simulink library "EqM"  (R2024a)
settings: Solver=VariableStepAuto  StartTime=0.0  StopTime=10.0  RelTol=1e-3
values from neighbouring files (symbols this model uses):
  g = 9.80665    [Initialization.m]    (also in Initialization_alt2.m; Initialization_cg1.m; Initialization_loop.m; Initialization_v2.m)
libraries: $bdroot x1
settings Model: Creator=Caê  LastModifiedBy=Caê
settings RTWCC: GPUComputeCapability=3.5

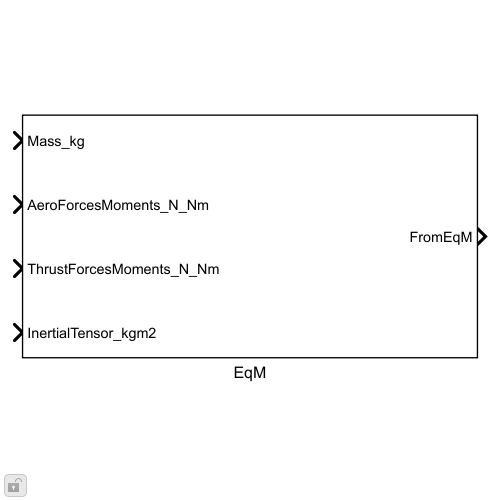
[thumbnail: Simulink's stored preview of the top-level diagram]
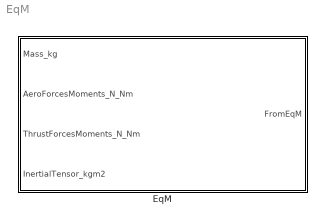
== system EqM ==
  EqM : Subsystem

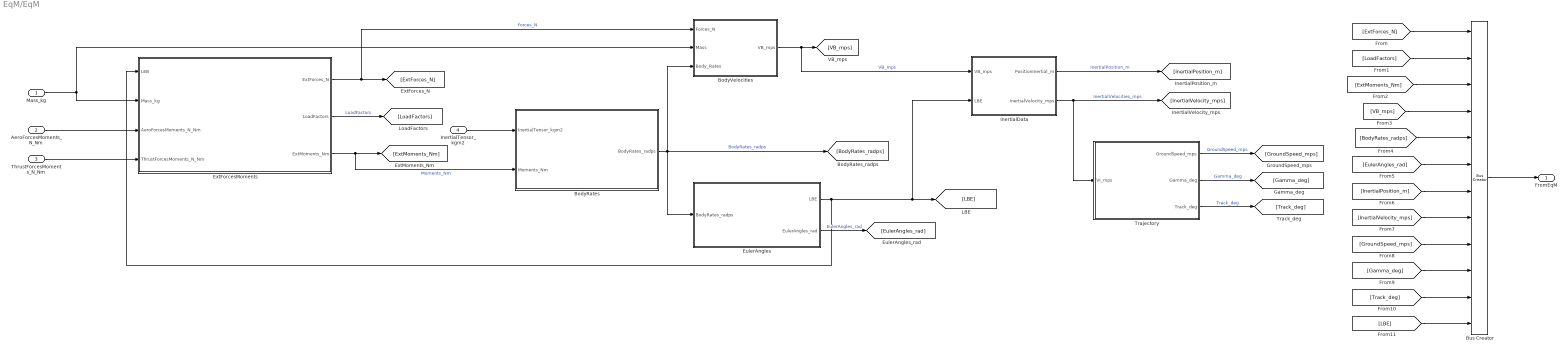
== system EqM/EqM ==
  Mass_kg : Inport
  AeroForcesMoments_N_Nm : Inport  Port=2
  ThrustForcesMoments_N_Nm : Inport  Port=3
  InertialTensor_kgm2 : Inport  Port=4
  BodyRates : Subsystem
  BodyVelocities : Subsystem
  Bus Creator : BusCreator  Inputs=12
  EulerAngles : Subsystem
  ExtForcesMoments : Subsystem
  InertialData : Subsystem
  Trajectory : Subsystem
  FromEqM : Outport
  wires:
  [LBE] -> Bus Creator/12
  [InertialPosition_m] -> Bus Creator/7
  ExtForcesMoments/3(ExtMoments_Nm) -> BodyRates/2(Moments_Nm), [ExtMoments_Nm]  "Moments_Nm"
  [EulerAngles_rad] -> Bus Creator/6
  [GroundSpeed_mps] -> Bus Creator/9
  Mass_kg/1 -> BodyVelocities/2(Mass), ExtForcesMoments/2(Mass_kg)
  ThrustForcesMoments_N_Nm/1 -> ExtForcesMoments/4(ThrustForcesMoments_N_Nm)
  InertialTensor_kgm2/1 -> BodyRates/1(InertialTensor_kgm2)
  [InertialVelocity_mps] -> Bus Creator/8
  [LoadFactors] -> Bus Creator/2
  InertialData/2(InertialVelocity_mps) -> [InertialVelocity_mps], Trajectory/1(VI_mps)  "InertialVelocities_mps"
  Bus Creator/1 -> FromEqM/1
  [BodyRates_radps] -> Bus Creator/5
  [Track_deg] -> Bus Creator/11
  EulerAngles/2(EulerAngles_rad) -> [EulerAngles_rad]  "EulerAngles_rad"
  [Gamma_deg] -> Bus Creator/10
  InertialData/1(PositionInertial_m) -> [InertialPosition_m]  "InertialPosition_m"
  ExtForcesMoments/2(LoadFactors) -> [LoadFactors]  "LoadFactors"
  BodyRates/1(BodyRates_radps) -> [BodyRates_radps], EulerAngles/1(BodyRates_radps), BodyVelocities/3(Body_Rates)  "BodyRates_radps"
  ExtForcesMoments/1(ExtForces_N) -> [ExtForces_N], BodyVelocities/1(Forces_N)  "Forces_N"
  BodyVelocities/1(VB_mps) -> [VB_mps], InertialData/1(VB_mps)  "VB_mps"
  [ExtMoments_Nm] -> Bus Creator/3
  AeroForcesMoments_N_Nm/1 -> ExtForcesMoments/3(AeroForcesMoments_N_Nm)
  Trajectory/1(GroundSpeed_mps) -> [GroundSpeed_mps]  "GroundSpeed_mps"
  [ExtForces_N] -> Bus Creator/1
  Trajectory/3(Track_deg) -> [Track_deg]  "Track_deg"
  EulerAngles/1(LBE) -> ExtForcesMoments/1(LEB), InertialData/2(LBE), [LBE]
  Trajectory/2(Gamma_deg) -> [Gamma_deg]  "Gamma_deg"
  [VB_mps] -> Bus Creator/4

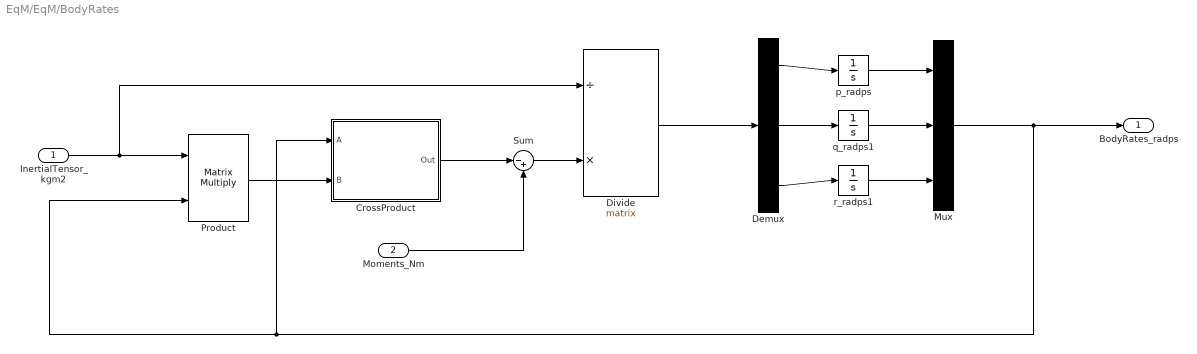
== system EqM/EqM/BodyRates ==
  InertialTensor_kgm2 : Inport
  Moments_Nm : Inport  Port=2
  CrossProduct : Subsystem
  Demux : Demux  Outputs=3
  Divide : Product  Inputs=/*  Multiplication=Matrix(*)
  Mux : Mux  Inputs=3
  Product : Product  Multiplication=Matrix(*)
  Sum : Sum  Inputs=|-+
  p_radps : Integrator  ContinuousStateAttributes='p_radps'
  q_radps1 : Integrator  ContinuousStateAttributes='q_radps'
  r_radps1 : Integrator  ContinuousStateAttributes='r_radps'
  BodyRates_radps : Outport
  wires:
  Demux/3 -> r_radps1/1
  InertialTensor_kgm2/1 -> Divide/1, Product/1
  Mux/1 -> BodyRates_radps/1, CrossProduct/1(A), Product/2
  q_radps1/1 -> Mux/2
  Sum/1 -> Divide/2
  Demux/1 -> p_radps/1
  Product/1 -> CrossProduct/2(B)
  p_radps/1 -> Mux/1
  CrossProduct/1(Out) -> Sum/1
  Moments_Nm/1 -> Sum/2
  r_radps1/1 -> Mux/3
  Demux/2 -> q_radps1/1
  Divide/1 -> Demux/1

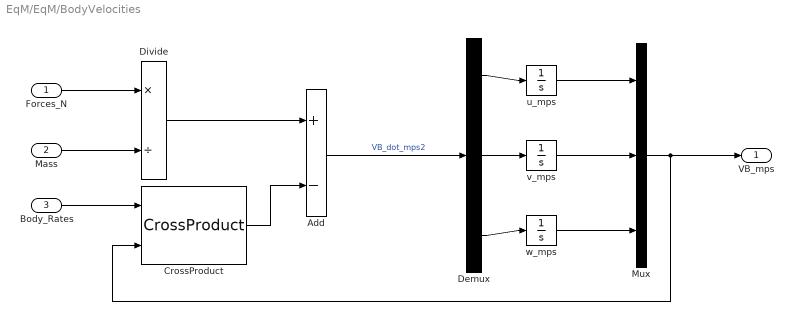
== system EqM/EqM/BodyVelocities ==
  Forces_N : Inport
  Mass : Inport  Port=2
  Body_Rates : Inport  Port=3
  Add : Sum  Inputs=+-
  CrossProduct : $bdroot/EqM/BodyRates/CrossProduct  SystemSampleTime=-1  VariantActivationTime=update diagram  AllowFlexibleInterface=on  Latency=0  AutoFrameSizeCalculation=off
  Demux : Demux  Outputs=3
  Divide : Product  Inputs=*/
  Mux : Mux  Inputs=3
  u_mps : Integrator  ContinuousStateAttributes='u_mps'
  v_mps : Integrator  ContinuousStateAttributes='v_mps'
  w_mps : Integrator  ContinuousStateAttributes='w_mps'
  VB_mps : Outport
  wires:
  CrossProduct/1 -> Add/2
  Demux/3 -> w_mps/1
  Mux/1 -> CrossProduct/2, VB_mps/1
  Forces_N/1 -> Divide/1
  Demux/2 -> v_mps/1
  u_mps/1 -> Mux/1
  Demux/1 -> u_mps/1
  Mass/1 -> Divide/2
  Body_Rates/1 -> CrossProduct/1
  Add/1 -> Demux/1  "VB_dot_mps2"
  w_mps/1 -> Mux/3
  v_mps/1 -> Mux/2
  Divide/1 -> Add/1

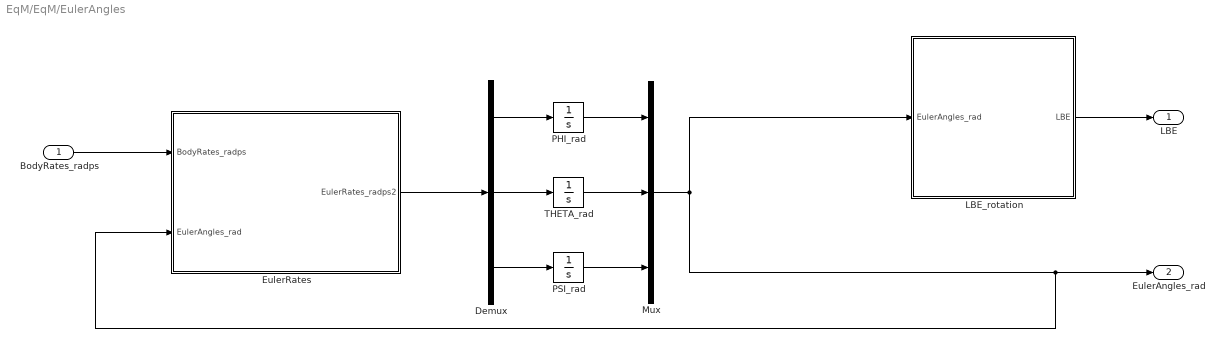
== system EqM/EqM/EulerAngles ==
  BodyRates_radps : Inport
  Demux : Demux  Outputs=3
  EulerRates : Subsystem
  LBE_rotation : Subsystem
  Mux : Mux  Inputs=3
  PHI_rad : Integrator  ContinuousStateAttributes='PHI_rad'
  PSI_rad : Integrator  ContinuousStateAttributes='PSI_rad'
  THETA_rad : Integrator  ContinuousStateAttributes='THETA_rad'
  LBE : Outport
  EulerAngles_rad : Outport  Port=2
  wires:
  Demux/3 -> PSI_rad/1
  Demux/2 -> THETA_rad/1
  Demux/1 -> PHI_rad/1
  PHI_rad/1 -> Mux/1
  Mux/1 -> EulerRates/2(EulerAngles_rad), EulerAngles_rad/1, LBE_rotation/1(EulerAngles_rad)
  PSI_rad/1 -> Mux/3
  EulerRates/1(EulerRates_radps2) -> Demux/1
  THETA_rad/1 -> Mux/2
  BodyRates_radps/1 -> EulerRates/1(BodyRates_radps)
  LBE_rotation/1(LBE) -> LBE/1

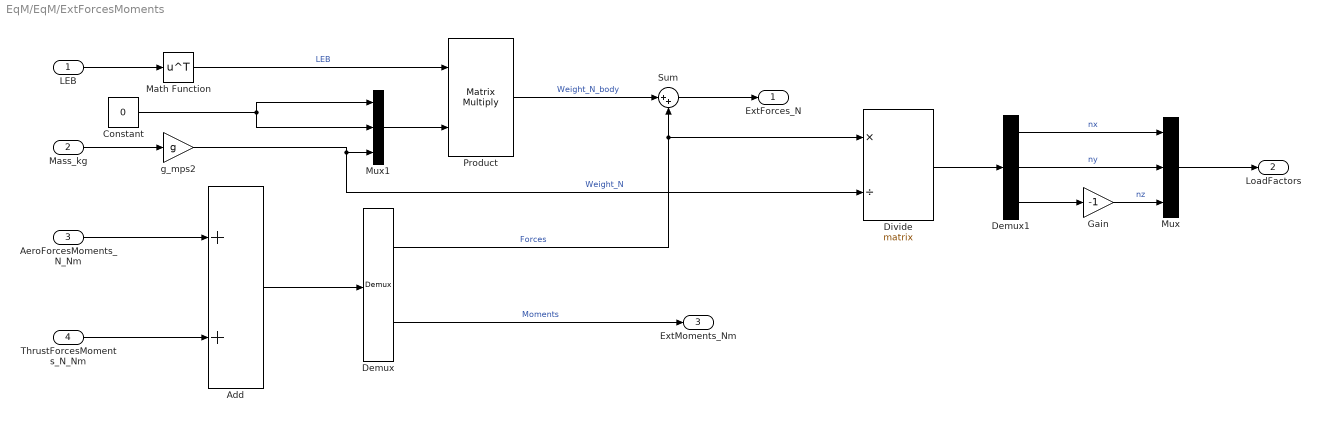
== system EqM/EqM/ExtForcesMoments ==
  LEB : Inport
  Mass_kg : Inport  Port=2
  AeroForcesMoments_N_Nm : Inport  Port=3
  ThrustForcesMoments_N_Nm : Inport  Port=4
  Add : Sum
  Constant : Constant  Value=0
  Demux : Demux  Outputs=2
  Demux1 : Demux  Outputs=3
  Divide : Product  Inputs=*/  Multiplication=Matrix(*)
  Gain : Gain  Gain=-1
  Math Function : Math  Operator=transpose
  Mux : Mux  Inputs=3
  Mux1 : Mux  Inputs=3
  Product : Product  Multiplication=Matrix(*)
  Sum : Sum  Inputs=|++
  g_mps2 : Gain  Gain=g
  ExtForces_N : Outport
  LoadFactors : Outport  Port=2
  ExtMoments_Nm : Outport  Port=3
  wires:
  Add/1 -> Demux/1
  Sum/1 -> ExtForces_N/1
  Mass_kg/1 -> g_mps2/1
  LEB/1 -> Math Function/1
  Demux/1 -> Divide/1, Sum/2  "Forces"
  Gain/1 -> Mux/3  "nz"
  Constant/1 -> Mux1/2, Mux1/1
  Math Function/1 -> Product/1  "LEB"
  g_mps2/1 -> Divide/2, Mux1/3  "Weight_N"
  Demux1/1 -> Mux/1  "nx"
  Product/1 -> Sum/1  "Weight_N_body"
  Demux1/2 -> Mux/2  "ny"
  Demux/2 -> ExtMoments_Nm/1  "Moments"
  Mux/1 -> LoadFactors/1
  AeroForcesMoments_N_Nm/1 -> Add/1
  Divide/1 -> Demux1/1
  ThrustForcesMoments_N_Nm/1 -> Add/2
  Demux1/3 -> Gain/1
  Mux1/1 -> Product/2

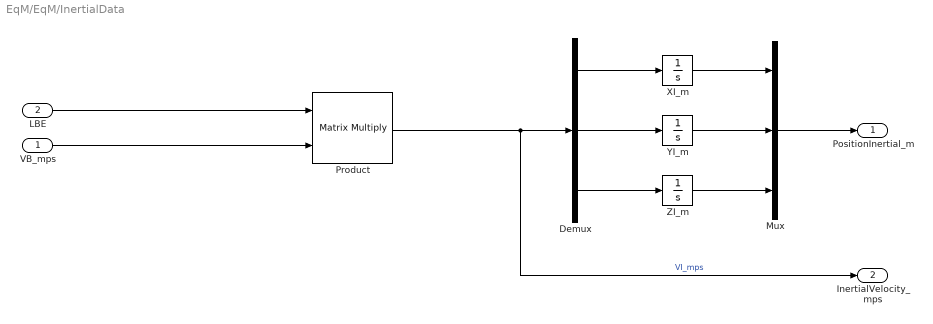
== system EqM/EqM/InertialData ==
  VB_mps : Inport
  LBE : Inport  Port=2
  Demux : Demux  Outputs=3
  Mux : Mux  Inputs=3
  Product : Product  Multiplication=Matrix(*)
  XI_m : Integrator  ContinuousStateAttributes='XI_m'
  YI_m : Integrator  ContinuousStateAttributes='YI_m'
  ZI_m : Integrator  ContinuousStateAttributes='ZI_m'
  PositionInertial_m : Outport
  InertialVelocity_mps : Outport  Port=2
  wires:
  Demux/1 -> XI_m/1
  ZI_m/1 -> Mux/3
  VB_mps/1 -> Product/2
  Product/1 -> InertialVelocity_mps/1, Demux/1  "VI_mps"
  XI_m/1 -> Mux/1
  Mux/1 -> PositionInertial_m/1
  YI_m/1 -> Mux/2
  Demux/3 -> ZI_m/1
  Demux/2 -> YI_m/1
  LBE/1 -> Product/1

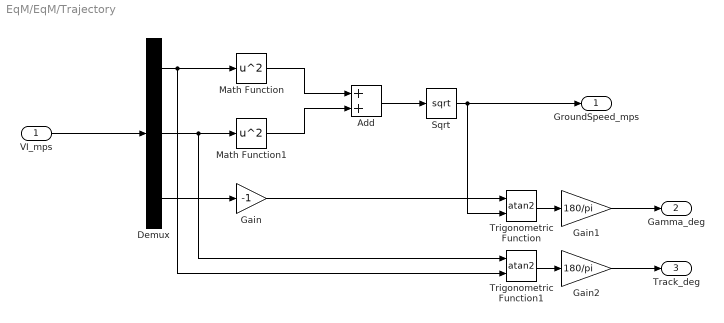
== system EqM/EqM/Trajectory ==
  VI_mps : Inport
  Add : Sum
  Demux : Demux  Outputs=3
  Gain : Gain  Gain=-1
  Gain1 : Gain  Gain=180/pi
  Gain2 : Gain  Gain=180/pi
  Math Function : Math  Operator=square
  Math Function1 : Math  Operator=square
  Sqrt : Sqrt
  Trigonometric Function : Trigonometry  Operator=atan2
  Trigonometric Function1 : Trigonometry  Operator=atan2
  GroundSpeed_mps : Outport
  Gamma_deg : Outport  Port=2
  Track_deg : Outport  Port=3
  wires:
  Sqrt/1 -> GroundSpeed_mps/1, Trigonometric Function/2
  Demux/1 -> Trigonometric Function1/2, Math Function/1
  Trigonometric Function/1 -> Gain1/1
  Demux/2 -> Trigonometric Function1/1, Math Function1/1
  VI_mps/1 -> Demux/1
  Add/1 -> Sqrt/1
  Trigonometric Function1/1 -> Gain2/1
  Gain/1 -> Trigonometric Function/1
  Demux/3 -> Gain/1
  Gain2/1 -> Track_deg/1
  Math Function1/1 -> Add/2
  Math Function/1 -> Add/1
  Gain1/1 -> Gamma_deg/1

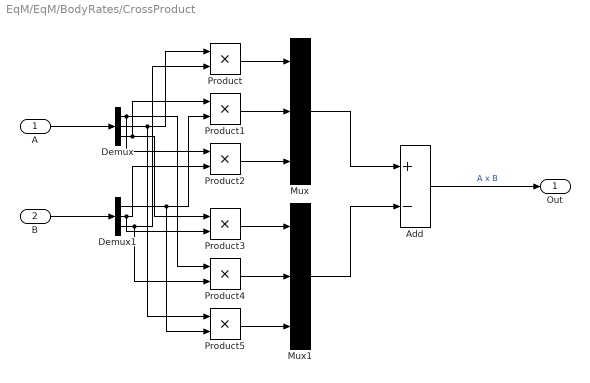
== system EqM/EqM/BodyRates/CrossProduct ==
  A : Inport
  B : Inport  Port=2
  Add : Sum  Inputs=+-
  Demux : Demux  Outputs=3
  Demux1 : Demux  Outputs=3
  Mux : Mux  Inputs=3
  Mux1 : Mux  Inputs=3
  Product{,1..5} (6 alike) : Product
  Out : Outport
  wires:
  Product5/1 -> Mux1/3
  Demux/2 -> Product5/1, Product/1
  Demux/1 -> Product4/1, Product2/1
  Mux/1 -> Add/1
  Product4/1 -> Mux1/2
  Product2/1 -> Mux/3
  Demux1/3 -> Product4/2, Product/2
  Demux/3 -> Product3/1, Product1/1
  Demux1/2 -> Product3/2, Product2/2
  Mux1/1 -> Add/2
  B/1 -> Demux1/1
  Product3/1 -> Mux1/1
  Product1/1 -> Mux/2
  Product/1 -> Mux/1
  Demux1/1 -> Product5/2, Product1/2
  A/1 -> Demux/1
  Add/1 -> Out/1  "A x B"

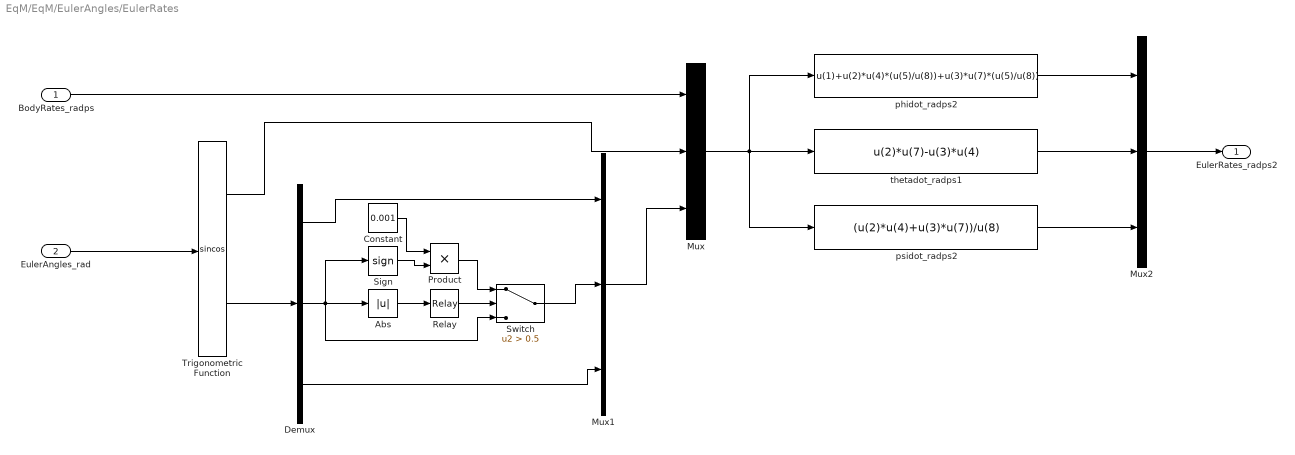
== system EqM/EqM/EulerAngles/EulerRates ==
  BodyRates_radps : Inport
  EulerAngles_rad : Inport  Port=2
  Abs : Abs  SaturateOnIntegerOverflow=off
  Constant : Constant  Value=0.001
  Demux : Demux  Outputs=3
  Mux : Mux  Inputs=3
  Mux1 : Mux  Inputs=3
  Mux2 : Mux  Inputs=3
  Product : Product
  Relay : Relay  OnSwitchValue=0.001  OffSwitchValue=0  OnOutputValue=0  OffOutputValue=1
  Sign : Signum
  Switch : Switch  Criteria=u2 > Threshold  Threshold=0.5  SaturateOnIntegerOverflow=off  InputSameDT=off
  Trigonometric Function : Trigonometry  Operator=sincos
  phidot_radps2 : Fcn  Expr=u(1)+u(2)*u(4)*(u(5)/u(8))+u(3)*u(7)*(u(5)/u(8))
  psidot_radps2 : Fcn  Expr=(u(2)*u(4)+u(3)*u(7))/u(8)
  thetadot_radps1 : Fcn  Expr=u(2)*u(7)-u(3)*u(4)
  EulerRates_radps2 : Outport
  wires:
  Demux/2 -> Sign/1, Abs/1, Switch/3
  Relay/1 -> Switch/2
  Demux/1 -> Mux1/1
  Abs/1 -> Relay/1
  Switch/1 -> Mux1/2
  Sign/1 -> Product/2
  Trigonometric Function/2 -> Demux/1
  Mux/1 -> psidot_radps2/1, phidot_radps2/1, thetadot_radps1/1
  phidot_radps2/1 -> Mux2/1
  BodyRates_radps/1 -> Mux/1
  Constant/1 -> Product/1
  Demux/3 -> Mux1/3
  EulerAngles_rad/1 -> Trigonometric Function/1
  Trigonometric Function/1 -> Mux/2
  thetadot_radps1/1 -> Mux2/2
  Mux1/1 -> Mux/3
  Product/1 -> Switch/1
  psidot_radps2/1 -> Mux2/3
  Mux2/1 -> EulerRates_radps2/1

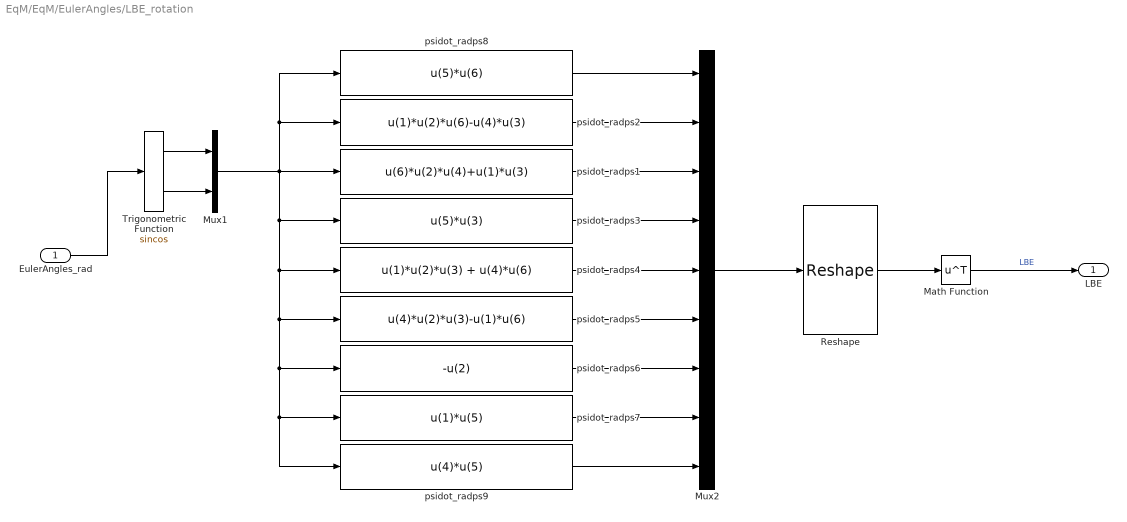
== system EqM/EqM/EulerAngles/LBE_rotation ==
  EulerAngles_rad : Inport
  Math Function : Math  Operator=transpose
  Mux1 : Mux  Inputs=2
  Mux2 : Mux  Inputs=9
  Reshape : Reshape  OutputDimensionality=Customize  OutputDimensions=[3,3]
  Trigonometric Function : Trigonometry  Operator=sincos
  psidot_radps1 : Fcn  Expr=u(6)*u(2)*u(4)+u(1)*u(3)
  psidot_radps2 : Fcn  Expr=u(1)*u(2)*u(6)-u(4)*u(3)
  psidot_radps3 : Fcn  Expr=u(5)*u(3)
  psidot_radps4 : Fcn  Expr=u(1)*u(2)*u(3) + u(4)*u(6)
  psidot_radps5 : Fcn  Expr=u(4)*u(2)*u(3)-u(1)*u(6)
  psidot_radps6 : Fcn  Expr=-u(2)
  psidot_radps7 : Fcn  Expr=u(1)*u(5)
  psidot_radps8 : Fcn  Expr=u(5)*u(6)
  psidot_radps9 : Fcn  Expr=u(4)*u(5)
  LBE : Outport
  wires:
  Mux2/1 -> Reshape/1
  psidot_radps9/1 -> Mux2/9
  Mux1/1 -> psidot_radps8/1, psidot_radps2/1, psidot_radps9/1, psidot_radps7/1, psidot_radps6/1, psidot_radps5/1, psidot_radps4/1, psidot_radps3/1, psidot_radps1/1
  Trigonometric Function/1 -> Mux1/1
  psidot_radps8/1 -> Mux2/1
  psidot_radps7/1 -> Mux2/8
  Reshape/1 -> Math Function/1
  psidot_radps5/1 -> Mux2/6
  Math Function/1 -> LBE/1  "LBE"
  EulerAngles_rad/1 -> Trigonometric Function/1
  Trigonometric Function/2 -> Mux1/2
  psidot_radps1/1 -> Mux2/3
  psidot_radps4/1 -> Mux2/5
  psidot_radps6/1 -> Mux2/7
  psidot_radps3/1 -> Mux2/4
  psidot_radps2/1 -> Mux2/2
